simulink model "wip"  (Simulink 7.9)
settings: Solver=ode45  StartTime=0.0  StopTime=50.0  RelTol=1e-3
undefined symbols (not defined in the file or in its folder): DiscIntNeverNeededParam
libraries: simulink x1
settings Model: Creator=dAN  LastModifiedBy=dAN

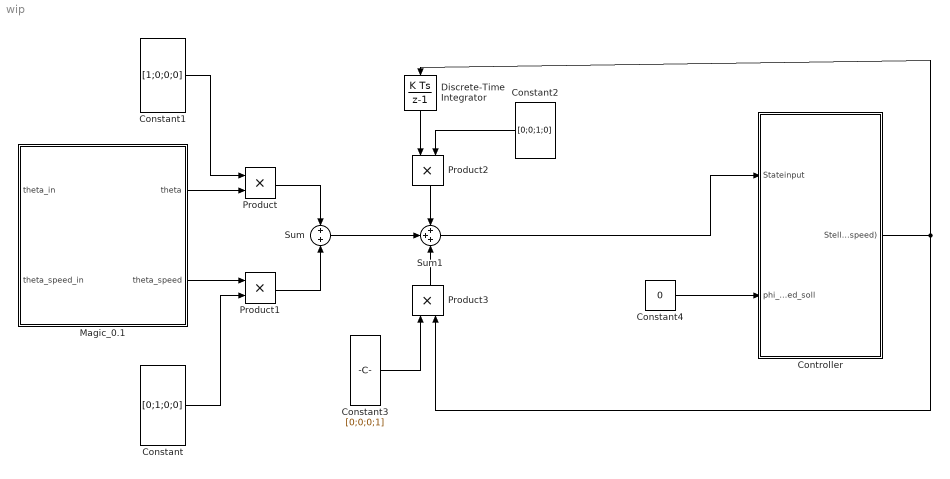
== system wip ==
  Constant : Constant  Value=[0;1;0;0]  VectorParams1D=off
  Constant1 : Constant  Value=[1;0;0;0]  VectorParams1D=off
  Constant2 : Constant  Value=[0;0;1;0]  VectorParams1D=off
  Constant3 : Constant  Value=[0;0;0;1]  VectorParams1D=off
  Constant4 : Constant  Value=0
  Controller : Subsystem
  Discrete-Time Integrator : DiscreteIntegrator  ICPrevOutput=DiscIntNeverNeededParam  ICPrevScaledInput=DiscIntNeverNeededParam
  Magic_0.1 : Subsystem
  Product{,1..3} (4 alike) : Product  RndMeth=Zero
  Sum : Sum  Inputs=+|+
  Sum1 : Sum  Inputs=+++
  wires:
  ? -> Magic_0.1/1(theta_in)
  ? -> Magic_0.1/2(theta_speed_in)
  Magic_0.1/1(theta) -> Product/2
  Magic_0.1/2(theta_speed) -> Product1/1
  Constant/1 -> Product1/2
  Constant1/1 -> Product/1
  Product/1 -> Sum/1
  Product1/1 -> Sum/2
  Controller/1(Stellgröße(phi_speed)) -> Discrete-Time Integrator/1, Product3/2
  Sum/1 -> Sum1/2
  Constant2/1 -> Product2/2
  Discrete-Time Integrator/1 -> Product2/1
  Constant3/1 -> Product3/1
  Sum1/1 -> Controller/1(Stateinput)
  Product2/1 -> Sum1/1
  Product3/1 -> Sum1/3
  Constant4/1 -> Controller/2(phi_speed_soll)

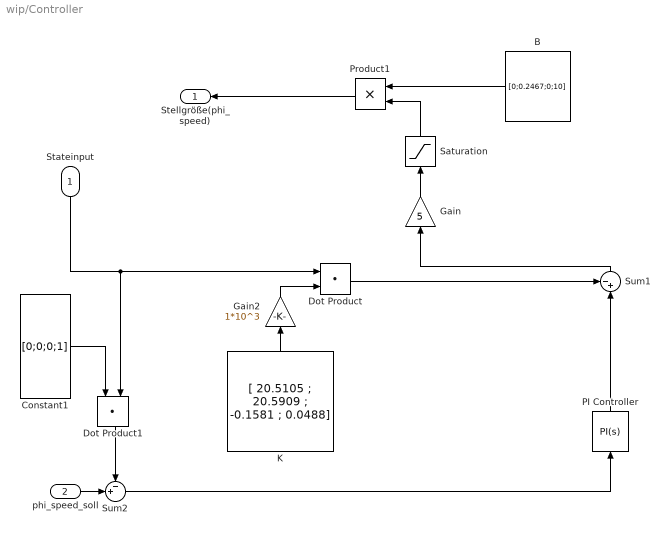
== system wip/Controller ==
  Stateinput : Inport
  phi_speed_soll : Inport  Port=2
  B : Constant  Value=[0;0.2467;0;10]  VectorParams1D=off
  Constant1 : Constant  Value=[0;0;0;1]  VectorParams1D=off
  Dot Product : DotProduct  InputSameDT=on  OutDataTypeStr=Inherit: Inherit via internal rule
  Dot Product1 : DotProduct  InputSameDT=on  OutDataTypeStr=Inherit: Inherit via internal rule
  Gain : Gain  Gain=5
  Gain2 : Gain  Gain=1*10^3
  K : Constant  Value="[ 20.5105 ;  20.5909 ;  -0.1581 ;   0.0488]"  VectorParams1D=off
  PI Controller : simulink/Continuous/PID Controller  Controller=PI  TimeDomain=Continuous-time  SampleTime=1  IntegratorMethod=Forward Euler  FilterMethod=Forward Euler  Form=Parallel  P=1  I=5  D=0  N=100  InitialConditionSource=internal  InitialConditionForIntegrator=0  InitialConditionForFilter=0  ExternalReset=none  LimitOutput=off  UpperSaturationLimit=inf  LowerSaturationLimit=-inf  LinearizeAsGain=off  AntiWindupMode=none  Kb=1  TrackingMode=off  Kt=1  PParamMin=[]  PParamMax=[]  IParamMin=[]  IParamMax=[]  DParamMin=[]  DParamMax=[]  NParamMin=[]  NParamMax=[]  KbParamMin=[]  KbParamMax=[]  KtParamMin=[]  KtParamMax=[]  POutMin=[]  POutMax=[]  IOutMin=[]  IOutMax=[]  DOutMin=[]  DOutMax=[]  NOutMin=[]  NOutMax=[]  KbOutMin=[]  KbOutMax=[]  KtOutMin=[]  KtOutMax=[]  IntegratorOutMin=[]  IntegratorOutMax=[]  FilterOutMin=[]  FilterOutMax=[]  SumOutMin=[]  SumOutMax=[]  SumI1OutMin=[]  SumI1OutMax=[]  SumI2OutMin=[]  SumI2OutMax=[]  SumI3OutMin=[]  SumI3OutMax=[]  SumDOutMin=[]  SumDOutMax=[]  SaturationOutMin=[]  SaturationOutMax=[]  IntegratorContinuousStateAttributes=''  IntegratorStateMustResolveToSignalObject=off  IntegratorRTWStateStorageClass=Auto  FilterContinuousStateAttributes=''  FilterStateMustResolveToSignalObject=off  FilterRTWStateStorageClass=Auto
  Product1 : Product  RndMeth=Zero
  Saturation : Saturate  UpperLimit=180  LowerLimit=-180
  Sum1 : Sum  Inputs=-+|
  Sum2 : Sum  Inputs=-+|
  Stellgröße(phi_speed) : Outport
  wires:
  phi_speed_soll/1 -> Sum2/2
  Stateinput/1 -> Dot Product1/2, Dot Product/1
  Product1/1 -> Stellgröße(phi_speed)/1
  Saturation/1 -> Product1/2
  PI Controller/1 -> Sum1/2
  Constant1/1 -> Dot Product1/1
  Gain2/1 -> Dot Product/2
  Dot Product1/1 -> Sum2/1
  Gain/1 -> Saturation/1
  Sum2/1 -> PI Controller/1
  Sum1/1 -> Gain/1
  Dot Product/1 -> Sum1/1
  B/1 -> Product1/1
  K/1 -> Gain2/1

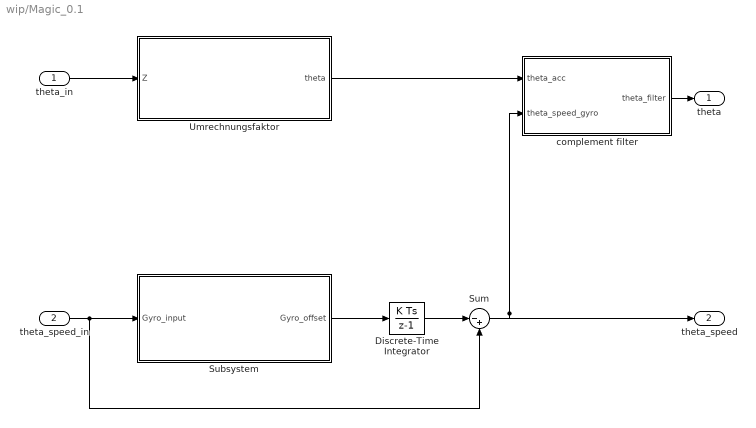
== system wip/Magic_0.1 ==
  theta_in : Inport
  theta_speed_in : Inport  Port=2
  Discrete-Time Integrator : DiscreteIntegrator  ICPrevOutput=DiscIntNeverNeededParam  ICPrevScaledInput=DiscIntNeverNeededParam
  Subsystem : Subsystem
  Sum : Sum  Inputs=|-+
  Umrechnungsfaktor : Subsystem
  complement filter : Subsystem
  theta : Outport
  theta_speed : Outport  Port=2
  wires:
  Umrechnungsfaktor/1(theta) -> complement filter/1(theta_acc)
  Subsystem/1(Gyro_offset) -> Discrete-Time Integrator/1
  Sum/1 -> complement filter/2(theta_speed_gyro), theta_speed/1
  Discrete-Time Integrator/1 -> Sum/1
  theta_speed_in/1 -> Subsystem/1(Gyro_input), Sum/2
  theta_in/1 -> Umrechnungsfaktor/1(Z)
  complement filter/1(theta_filter) -> theta/1

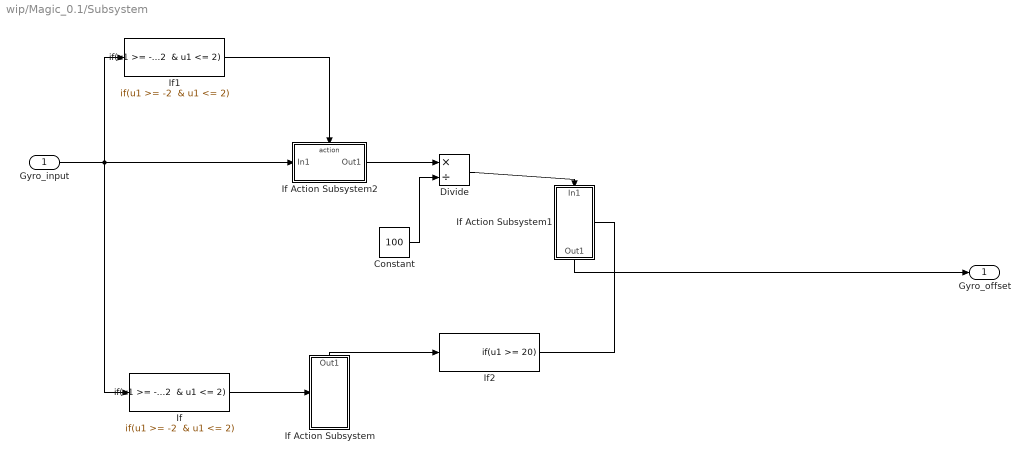
== system wip/Magic_0.1/Subsystem ==
  Gyro_input : Inport
  Constant : Constant  Value=100
  Divide : Product  Inputs=*/
  If : If  IfExpression="u1 >= -2  & u1 <= 2"  ShowElse=off
  If Action Subsystem : Subsystem  TreatAsAtomicUnit=on
  If Action Subsystem1 : Subsystem  TreatAsAtomicUnit=on
  If Action Subsystem2 : Subsystem  TreatAsAtomicUnit=on
  If1 : If  IfExpression="u1 >= -2  & u1 <= 2"  ShowElse=off
  If2 : If  IfExpression=u1 >= 20  ShowElse=off
  Gyro_offset : Outport
  wires:
  Gyro_input/1 -> If/1, If Action Subsystem2/1(In1), If1/1
  If/1 -> If Action Subsystem/Action
  If Action Subsystem/1(Out1) -> If2/1
  If Action Subsystem2/1(Out1) -> Divide/1
  Divide/1 -> If Action Subsystem1/1(In1)
  Constant/1 -> Divide/2
  If1/1 -> If Action Subsystem2/Action
  If2/1 -> If Action Subsystem1/Action
  If Action Subsystem1/1(Out1) -> Gyro_offset/1

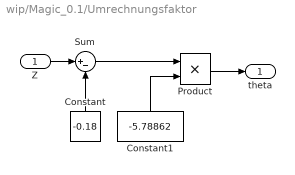
== system wip/Magic_0.1/Umrechnungsfaktor ==
  Z : Inport
  Constant : Constant  Value=-0.18
  Constant1 : Constant  Value=-5.78862
  Product : Product  RndMeth=Zero
  Sum : Sum  Inputs=|+-
  theta : Outport
  wires:
  Constant/1 -> Sum/2
  Sum/1 -> Product/1
  Constant1/1 -> Product/2
  Z/1 -> Sum/1
  Product/1 -> theta/1

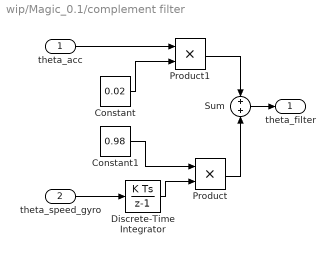
== system wip/Magic_0.1/complement filter ==
  theta_acc : Inport
  theta_speed_gyro : Inport  Port=2
  Constant : Constant  Value=0.02
  Constant1 : Constant  Value=0.98
  Discrete-Time Integrator : DiscreteIntegrator  ICPrevOutput=DiscIntNeverNeededParam  ICPrevScaledInput=DiscIntNeverNeededParam
  Product : Product  RndMeth=Zero
  Product1 : Product  RndMeth=Zero
  Sum : Sum  Inputs=+|+
  theta_filter : Outport
  wires:
  Product1/1 -> Sum/1
  Product/1 -> Sum/2
  Constant/1 -> Product1/2
  Constant1/1 -> Product/1
  Discrete-Time Integrator/1 -> Product/2
  theta_acc/1 -> Product1/1
  Sum/1 -> theta_filter/1
  theta_speed_gyro/1 -> Discrete-Time Integrator/1

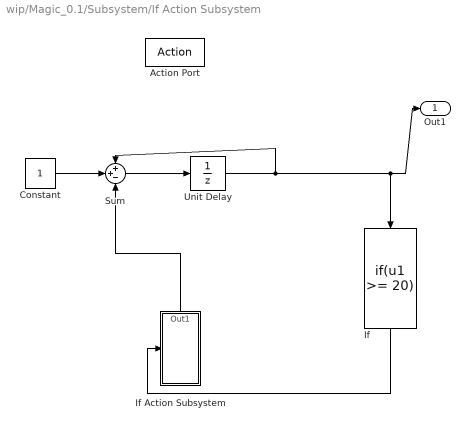
== system wip/Magic_0.1/Subsystem/If Action Subsystem ==
  Action Port : ActionPort  ActionType=then
  Constant : Constant
  If : If  IfExpression=u1 >= 20  ShowElse=off
  If Action Subsystem : Subsystem  TreatAsAtomicUnit=on
  Sum : Sum  Inputs=++-
  Unit Delay : UnitDelay  SampleTime=-1
  Out1 : Outport
  wires:
  Unit Delay/1 -> Sum/1, Out1/1, If/1
  If Action Subsystem/1(Out1) -> Sum/3
  Sum/1 -> Unit Delay/1
  Constant/1 -> Sum/2
  If/1 -> If Action Subsystem/Action

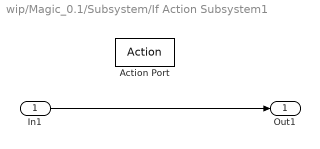
== system wip/Magic_0.1/Subsystem/If Action Subsystem1 ==
  In1 : Inport
  Action Port : ActionPort  ActionType=then
  Out1 : Outport
  wires:
  In1/1 -> Out1/1

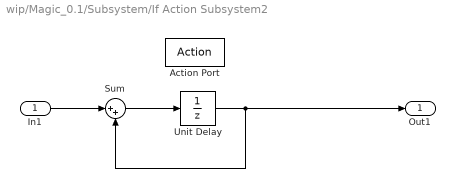
== system wip/Magic_0.1/Subsystem/If Action Subsystem2 ==
  In1 : Inport
  Action Port : ActionPort  ActionType=then
  Sum : Sum  Inputs=|++
  Unit Delay : UnitDelay  SampleTime=-1
  Out1 : Outport
  wires:
  In1/1 -> Sum/1
  Sum/1 -> Unit Delay/1
  Unit Delay/1 -> Sum/2, Out1/1

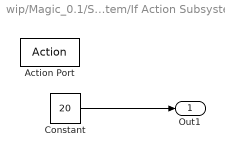
== system wip/Magic_0.1/Subsystem/If Action Subsystem/If Action Subsystem ==
  Action Port : ActionPort  ActionType=then
  Constant : Constant  Value=20
  Out1 : Outport
  wires:
  Constant/1 -> Out1/1
